simulink model "cc"  (R2021a)
settings: Solver=VariableStepAuto  StartTime=0.0  StopTime=10  RelTol=1e-3
libraries: spsSeriesRLCBranchLib x4, spsCurrentMeasurementLib x1, spsPWMGeneratorDCDCLib x1, spsPVArrayLib x1, spsVoltageMeasurementLib x1, spsDiodeLib x1, spsMosfetLib x1, spspowerguiLib x1
settings Model: Creator=mluser  LastModifiedBy=mluser
settings SolverCC: AlgebraicLoopSolver=TrustRegion
settings DebuggingCC: SFMachineParentedDataDiag=warning

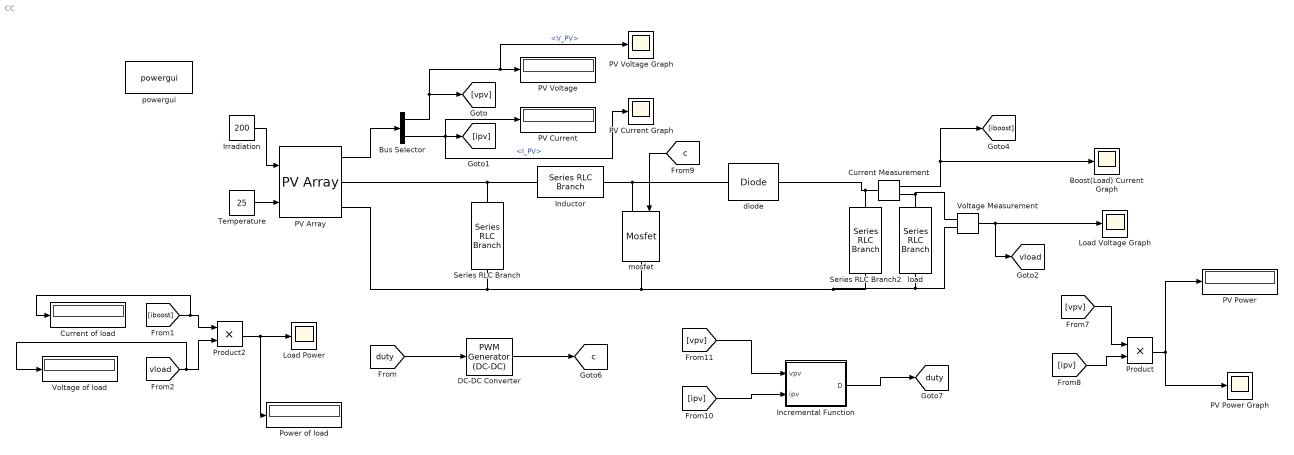
== system cc ==
  Boost(Load) Current Graph : Scope
  Bus Selector : BusSelector  OutputSignals=V_PV,I_PV
  Current Measurement : spsCurrentMeasurementLib/Current Measurement  PhasorSimulation=off  OutputType=Complex  PSBequivalent=0
  Current of load : Display
  DC-DC Converter : spsPWMGeneratorDCDCLib/PWM Generator (DC-DC)  Fsw=5000  Ts=0
  Incremental Function : MATLAB Function  TreatAsAtomicUnit=on
  Inductor : spsSeriesRLCBranchLib/Series RLC Branch  LConnTagsString=__new0  RConnTagsString=__new0  BranchType=L  Resistance=0.1  Inductance=1e-3  SetiL0=off  InitialCurrent=0  Capacitance=1e-6  Setx0=off  InitialVoltage=0  Measurements=None
  Irradiation : Constant  Value=200
  Load Power : Scope
  Load Voltage Graph : Scope
  PV Array : spsPVArrayLib/PV Array  Npar=5  Nser=1  PlotType=array @ 1000 W/m2 & specified temperatures  S_vec="[ 1000  500  100 ]"  Temp_C_vec="[ 45 25  ]"  ModuleName=User-defined  PlotWhenSelected=off  Pm=213.15  Ncell=36  Voc=36.3  Isc=7.84  Vm=29  Im=7.35  beta_Voc_pc=-0.36099  alpha_Isc_pc=0.102  beta_Voc=-0.13104  alpha_Isc=0.0079968  IL=7.8922  I0=2.8997e-10  nI=1.6349  Rsh=220.9676  Rs=0.39348  RobustModel=off  RobustCellTemperature=313.3991  BAL=on  Tc=1e-6  Tfilter=5e-5
  PV Current : Display
  PV Current Graph : Scope
  PV Power : Display
  PV Power Graph : Scope
  PV Voltage : Display
  PV Voltage Graph : Scope
  Power of load : Display
  Product : Product
  Product2 : Product
  Series RLC Branch : spsSeriesRLCBranchLib/Series RLC Branch  LConnTagsString=__new0  RConnTagsString=__new0  BranchType=RC  Resistance=1e-4  Inductance=1e-3  SetiL0=off  InitialCurrent=0  Capacitance=100e-6  Setx0=off  InitialVoltage=0  Measurements=None
  Series RLC Branch2 : spsSeriesRLCBranchLib/Series RLC Branch  LConnTagsString=__new0  RConnTagsString=__new0  BranchType=C  Resistance=1e-4  Inductance=1e-3  SetiL0=off  InitialCurrent=0  Capacitance=3300e-6  Setx0=off  InitialVoltage=0  Measurements=None
  Temperature : Constant  Value=25
  Voltage Measurement : spsVoltageMeasurementLib/Voltage Measurement  PhasorSimulation=off  OutputType=Complex  PSBequivalent=0
  Voltage of load : Display
  diode : spsDiodeLib/Diode  Ron=0.001  Lon=0  Vf=0.8  IC=0  UseSnubber=0  Rs=500  Cs=250e-9  Measurements=off
  load : spsSeriesRLCBranchLib/Series RLC Branch  LConnTagsString=__new0  RConnTagsString=__new0  BranchType=R  Resistance=500  Inductance=1e-3  SetiL0=off  InitialCurrent=0  Capacitance=3300e-6  Setx0=off  InitialVoltage=0  Measurements=None
  mosfet : spsMosfetLib/Mosfet  Ron=0.001  Lon=0  Rd=0.001  Vfd=0  IC=0  Rs=1e5  Cs=inf  Measurements=off
  powergui : spspowerguiLib/powergui  Priority=1  SimulationMode=Discrete  SampleTime=10e-6  frequency=60  Iterations=50  frequencyindice=0  Pbase=100e6  ErrMax=1e-4  UnitsV=kV  UnitsW=MW  buscounter=0  FunctionMessages=off  echomessages=off  EnableUseOfTLC=off  CurrentSourceSwitches=off  DisableSnubberDevices=off  DisableRonSwitches=off  DisableVfSwitches=off  DisplayEquations=off  AutomaticDiscreteSolvers=off  SolverType=Tustin/Backward Euler (TBE)  Interpol=off  ExternalGateDelay=off  methode=off  Ts=100  x0status=blocks  SPID=on  SwTol=0  HookPort=off  NonlinearTolerance=1e-4  nMaxIteration=100  ContinueOnMaxIteration=off  RestoreLinks=warning  ResistiveCurrentMeasurement=off  Frange=[0:2:500]  Ylog=off  Xlog=on  ShowGrid=off  save=off  variable=ZData  structure=0  ZoomFFT=off  StartTime=0.0  cycles=1  DisplayStyle=1  fundamental=60  FreqAxis=off  MaxFrequency=1000  frequencyindicesteady=1  RmsSteady=1  display=off
  tag scope: c=global, duty=global, vload=global
  wires:
  PV Array/1 -> Bus Selector/1
  Bus Selector/1 -> PV Voltage Graph/1, PV Voltage/1, [vpv]  "<V_PV>"
  Bus Selector/2 -> PV Current Graph/1, PV Current/1, [ipv]  "<I_PV>"
  Irradiation/1 -> PV Array/1
  Temperature/1 -> PV Array/2
  Voltage Measurement/1 -> [vload], Load Voltage Graph/1
  Current Measurement/1 -> Boost(Load) Current Graph/1, [iboost]
  [ipv] -> Product/2
  [vpv] -> Product/1
  Product/1 -> PV Power/1, PV Power Graph/1
  [duty] -> DC-DC Converter/1
  DC-DC Converter/1 -> [c]
  [ipv] -> Incremental Function/2(ipv)
  [c] -> mosfet/1
  [iboost] -> Current of load/1, Product2/1
  [vload] -> Voltage of load/1, Product2/2
  Product2/1 -> Power of load/1, Load Power/1
  [vpv] -> Incremental Function/1(vpv)
  Incremental Function/1(D) -> [duty]
  connections:
  PV Array/RConn1 -- Series RLC Branch/LConn1 -- Inductor/LConn1
  PV Array/RConn2 -- Voltage Measurement/LConn2 -- load/RConn1 -- Series RLC Branch2/RConn1 -- mosfet/RConn1 -- Series RLC Branch/RConn1
  diode/LConn1 -- mosfet/LConn1 -- Inductor/RConn1
  diode/RConn1 -- Current Measurement/LConn1 -- Series RLC Branch2/LConn1
  load/LConn1 -- Current Measurement/RConn1 -- Voltage Measurement/LConn1

== matlab function cc/Incremental Function ==
  data: vpv input; ipv input; D output
function D = Increm(vpv, ipv)

persistent Do Io Vo

dataType = 'double';

if isempty(Vo)
    Do = 0.7;
    Vo = 190;
    Io = 10.5;
end

deltaD=125e-6;
dv=vpv-Vo;
di=ipv-Io;
if dv==0
    if di==0
        D=Do;
    else
        if di>0
            D=Do-deltaD;
        else
            D= Do+deltaD;
        end
    end
else 
    if di/dv == -(ipv/vpv)
        D= Do;
else
    if di/dv > -(ipv/vpv)
    D=Do-deltaD;
else
    D= Do+deltaD;
end
end
    
end

Do=D;
Io=ipv;
Vo=vpv;
